simulink model "gm_sampleModel1853_5_sub"  (R2023a)
settings: Solver=VariableStepAuto  StartTime=0.0  StopTime=10.0  RelTol=1e-3
libraries: simulink x3, hdlsllib x2
settings Model: Creator=user1  LastModifiedBy=user1
settings OptimizationCC: BlockReduction=off  ConditionallyExecuteInputs=off
settings DebuggingCC: InheritedTsInSrcMsg=none

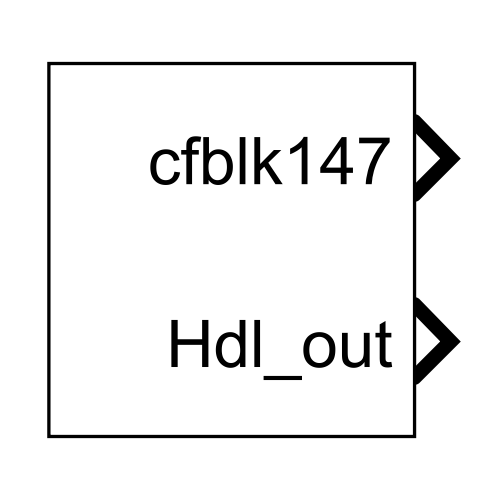
[thumbnail: Simulink's stored preview of the top-level diagram]
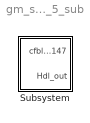
== system gm_sampleModel1853_5_sub ==
  Subsystem : Subsystem

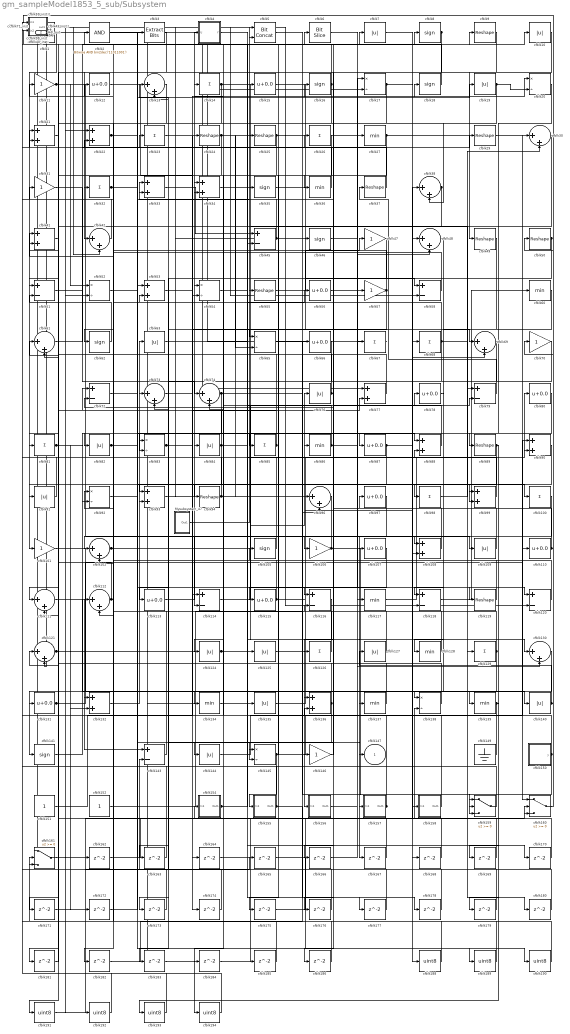
== system gm_sampleModel1853_5_sub/Subsystem ==
  Mysubsystem_47 : Subsystem
  cfblk1 : simulink/Logic and Bit Operations/Detect Increase  vinit=0.0  OutDataTypeStr=uint8
      settings: LibrarySourceBlock=|
      | hdlsllib/Logic and Bit
      | Operations/Detect
      | Increase
  cfblk{7,10,19,63,76,82,84,91,109,124..125,127,135,140,144} (15 alike) : Abs  OutDataTypeStr=uint8  SaturateOnIntegerOverflow=off
  cfblk{14,23,26,32,67..68,81,85,98,100,126,129} (12 alike) : Sum  Inputs=+  OutDataTypeStr=uint8
  cfblk{11,31,47,57,70,101,106,146} (8 alike) : Gain  OutDataTypeStr=uint8
  cfblk{13,30,38,42,48,61,69,73..74,96,102,111..112,121,130} (15 alike) : Sum  Inputs=|++  OutDataTypeStr=uint8
  cfblk103_inst : Subsystem
  cfblk104_inst : Subsystem
  cfblk{8,16,18,35,46,62,105,141} (8 alike) : Signum
  cfblk{12,15,56,66,78,80,87,97,107,110,113,115,131} (13 alike) : Bias  Bias=0.0  SaturateOnIntegerOverflow=off
  cfblk{21..22,33..34,41,53,77,88,90,93,99,108,132,136} (14 alike) : Sum  OutDataTypeStr=uint8
  cfblk{45,51,58,72,79,114,116,118,120,143} (10 alike) : Sum  Inputs=+-  OutDataTypeStr=uint8
  cfblk{27,36,60,86,117,128,134,137,139} (9 alike) : MinMax  OutDataTypeStr=uint8
  cfblk{9,24..25,29,37,49..50,55,89,94,119} (11 alike) : Reshape
  cfblk122_inst : Subsystem
  cfblk123_inst : Subsystem
  cfblk133_inst : Subsystem
  cfblk{17,20,52,54,65,83,92,138,145} (9 alike) : Product  Inputs=*/  OutDataTypeStr=uint8  RndMeth=Zero  SaturateOnIntegerOverflow=on
  cfblk142_inst : Subsystem
  cfblk149 : Ground
  cfblk150 : Subsystem  mask(Counter Limited){uplimit=double(7), tsamp=double(-1)}
      mask prompts: uplimit "Simulink:masks:UpperLimit_MP"; tsamp "Simulink:masks:SampleTime_MP"
      mask help: Simulink:masks:CounterLimited_MD
      mask init:
      | nbits = double(8);
      | tsamp = double(-1);
      | uplimit = double(7);
  cfblk151 : Constant  OutDataTypeStr=uint8  SampleTime=-1
  cfblk152 : Constant  OutDataTypeStr=uint8  SampleTime=-1
  cfblk154 : Subsystem
  cfblk155 : Subsystem
  cfblk156 : Subsystem
  cfblk157 : Subsystem
  cfblk158 : Subsystem
  cfblk159 : Switch  OutDataTypeStr=uint8  SaturateOnIntegerOverflow=off  InputSameDT=off
  cfblk160 : Switch  OutDataTypeStr=uint8  SaturateOnIntegerOverflow=off  InputSameDT=off
  cfblk161 : Switch  OutDataTypeStr=uint8  SaturateOnIntegerOverflow=off  InputSameDT=off
  cfblk{162..186} (25 alike) : Delay  SampleTime=1
  cfblk{188..194} (7 alike) : DataTypeConversion  OutDataTypeStr=uint8  SaturateOnIntegerOverflow=off  RndMeth=Floor
  cfblk2 : simulink/Logic and Bit Operations/Bitwise Operator  logicop=AND  UseBitMask=on  BitMask=bin2dec('11011001')  BitMaskRealWorld=Stored Integer
      settings: LibrarySourceBlock=|
      | hdlsllib/Logic and Bit
      | Operations/Bitwise
      | Operator
  cfblk28_inst : Subsystem
  cfblk3 : simulink/Logic and Bit Operations/Extract Bits  bitsToExtract=Upper half  numBits=8  bitIdxRange=[0 7]  outScalingMode=Preserve fixed-point scaling
      settings: LibrarySourceBlock=|
      | hdlsllib/Logic and Bit
      | Operations/Extract Bits
  cfblk39_inst : Subsystem
  cfblk4 : Subsystem  mask(Detect Fall Nonpositive){vinit=double(0), InputProcessing=Elements as channels (sample based), OutDataTypeStr=uint8}
      mask prompts: vinit "Simulink:masks:InitialCondition_MP"; InputProcessing "Simulink:masks:InputProcessing_MP"; OutDataTypeStr "Simulink:masks:OutputDataType_MP"
      mask help: Simulink:masks:DetectFallNonpositive_MD
      mask init:
      | InputProcessing = 'Elements as channels (sample based)';
      | OutDataTypeStr = 'uint8';
      | vinit = double(0);
      mask TypeOptions InputProcessing: Simulink:masks:ColumnsAsChannelsFrameBased | Simulink:masks:ElementsAsChannelsSampleBased
      mask TypeOptions OutDataTypeStr: Simulink:masks:uint8 | Simulink:masks:boolean
      mask Display: fprintf('U <= 0\n&  NOT\nU/z <= 0')
  cfblk40_inst : Subsystem
  cfblk43_inst : Subsystem
  cfblk5 : hdlsllib/Logic and Bit Operations/Bit Concat  numInputs=2
  cfblk59_inst : Subsystem
  cfblk6 : hdlsllib/Logic and Bit Operations/Bit Slice  lidx=7  ridx=0
  cfblk71_inst : Subsystem
  cfblk95_inst : Subsystem
  cfblk147 : Outport  OutDataTypeStr=uint8  SampleTime=1  VectorParamsAs1DForOutWhenUnconnected=off
  Hdl_out : Outport  Port=2  OutDataTypeStr=uint8
  wires:
  Mysubsystem_47/1(Out1) -> cfblk5/1
  cfblk1/1 -> cfblk101/1
  cfblk10/1 -> cfblk49/1
  cfblk100/1 -> cfblk167/1
  cfblk101/1 -> cfblk139/1
  cfblk102/1 -> cfblk76/1, cfblk120/1
  cfblk103_inst/1(out1) -> cfblk42/2, cfblk135/1
  cfblk104_inst/1(out1) -> cfblk125/1
  cfblk105/1 -> cfblk63/1
  cfblk106/1 -> cfblk159/3, cfblk102/1
  cfblk107/1 -> cfblk145/2
  cfblk108/1 -> cfblk97/1
  cfblk109/1 -> cfblk33/1
  cfblk11/1 -> cfblk114/2, cfblk52/1
  cfblk110/1 -> cfblk95_inst/1(in1), cfblk72/2, cfblk107/1
  cfblk111/1 -> cfblk143/1
  cfblk112/1 -> cfblk61/1, cfblk92/1
  cfblk113/1 -> cfblk4/1(U)
  cfblk114/1 -> cfblk78/1
  cfblk115/1 -> cfblk88/2, cfblk11/1
  cfblk116/1 -> cfblk156/1(In1)
  cfblk117/1 -> cfblk80/1
  cfblk118/1 -> cfblk60/1
  cfblk119/1 -> cfblk53/2
  cfblk12/1 -> cfblk174/1
  cfblk120/1 -> cfblk41/1
  cfblk121/1 -> cfblk66/1, cfblk132/2
  cfblk122_inst/1(out1) -> cfblk77/1, cfblk58/2
  cfblk123_inst/1(out1) -> cfblk96/1
  cfblk124/1 -> cfblk90/2, cfblk18/1
  cfblk125/1 -> cfblk68/1
  cfblk126/1 -> cfblk54/1
  cfblk127/1 -> cfblk84/1, cfblk21/1
  cfblk128/1 -> cfblk114/1
  cfblk129/1 -> cfblk157/1(In1), cfblk23/1
  cfblk13/1 -> cfblk191/1
  cfblk130/1 -> cfblk141/1
  cfblk131/1 -> cfblk90/1, cfblk3/1
  cfblk132/1 -> cfblk73/1
  cfblk133_inst/1(out1) -> cfblk30/1
  cfblk134/1 -> cfblk20/1
  cfblk135/1 -> cfblk57/1
  cfblk136/1 -> cfblk93/2, cfblk173/1
  cfblk137/1 -> cfblk122_inst/2(in2)
  cfblk138/1 -> cfblk6/1
  cfblk139/1 -> cfblk193/1, cfblk136/2
  cfblk14/1 -> cfblk42/1, cfblk137/1
  cfblk140/1 -> cfblk127/1, cfblk70/1
  cfblk141/1 -> cfblk112/1
  cfblk142_inst/1(out1) -> cfblk161/1, cfblk52/2
  cfblk143/1 -> cfblk28_inst/1(in1)
  cfblk144/1 -> cfblk110/1
  cfblk145/1 -> cfblk38/1, cfblk105/1, cfblk155/1(In1)
  cfblk146/1 -> cfblk86/1
  cfblk149/1 -> cfblk71_inst/2(in2)
  cfblk15/1 -> cfblk58/1
  cfblk150/1(y) -> cfblk5/2, cfblk159/2, cfblk116/2
  cfblk151/1 -> cfblk24/1
  cfblk152/1 -> cfblk45/2
  cfblk154/1(Out1) -> cfblk8/1, cfblk16/1, cfblk10/1
  cfblk155/1(Out1) -> cfblk43_inst/2(in2), cfblk177/1
  cfblk156/1(Out1) -> cfblk117/1
  cfblk157/1(Out1) -> cfblk74/2, cfblk13/1
  cfblk158/1(Out1) -> cfblk55/1
  cfblk159/1 -> cfblk122_inst/1(in1)
  cfblk16/1 -> cfblk132/1, cfblk103_inst/1(in1)
  cfblk160/1 -> cfblk50/1
  cfblk161/1 -> cfblk154/1(In1)
  cfblk162/1 -> cfblk160/2
  cfblk163/1 -> cfblk142_inst/2(in2)
  cfblk164/1 -> cfblk17/1
  cfblk165/1 -> cfblk190/1
  cfblk166/1 -> cfblk130/2
  cfblk167/1 -> cfblk111/2
  cfblk168/1 -> cfblk73/2
  cfblk169/1 -> cfblk121/1
  cfblk17/1 -> cfblk69/2, cfblk146/1
  cfblk170/1 -> cfblk138/2
  cfblk171/1 -> cfblk160/3
  cfblk172/1 -> cfblk34/1
  cfblk173/1 -> cfblk28_inst/2(in2)
  cfblk174/1 -> cfblk53/1
  cfblk175/1 -> cfblk118/2
  cfblk176/1 -> cfblk112/2
  cfblk177/1 -> cfblk33/2
  cfblk178/1 -> cfblk143/2
  cfblk179/1 -> cfblk40_inst/2(in2)
  cfblk18/1 -> cfblk133_inst/2(in2)
  cfblk180/1 -> cfblk161/2
  cfblk181/1 -> cfblk61/2
  cfblk182/1 -> cfblk96/2
  cfblk183/1 -> cfblk194/1
  cfblk184/1 -> cfblk48/1
  cfblk185/1 -> cfblk102/2
  cfblk186/1 -> cfblk161/3
  cfblk188/1 -> cfblk2/1
  cfblk189/1 -> cfblk71_inst/1(in1)
  cfblk19/1 -> cfblk82/1, cfblk38/2, cfblk20/2
  cfblk190/1 -> cfblk123_inst/2(in2)
  cfblk191/1 -> cfblk165/1
  cfblk192/1 -> cfblk123_inst/1(in1)
  cfblk193/1 -> cfblk39_inst/1(in1)
  cfblk194/1 -> cfblk39_inst/2(in2)
  cfblk2/1 -> cfblk189/1
  cfblk20/1 -> cfblk89/1
  cfblk21/1 -> cfblk181/1
  cfblk22/1 -> cfblk9/1, cfblk19/1
  cfblk23/1 -> cfblk164/1
  cfblk24/1 -> cfblk188/1, cfblk65/2, cfblk54/2
  cfblk25/1 -> cfblk51/1, cfblk111/1
  cfblk26/1 -> cfblk144/1
  cfblk27/1 -> cfblk65/1, cfblk166/1
  cfblk28_inst/1(out1) -> cfblk121/2, cfblk120/2, cfblk185/1
  cfblk29/1 -> cfblk160/1
  cfblk3/1 -> cfblk32/1
  cfblk30/1 -> cfblk81/1
  cfblk31/1 -> cfblk74/1
  cfblk32/1 -> cfblk87/1, cfblk147/1
  cfblk33/1 -> cfblk45/1
  cfblk34/1 -> cfblk129/1
  cfblk35/1 -> cfblk168/1
  cfblk36/1 -> cfblk40_inst/1(in1)
  cfblk37/1 -> cfblk14/1
  cfblk38/1 -> cfblk62/1, cfblk175/1
  cfblk39_inst/1(out1) -> cfblk192/1
  cfblk4/1(Y) -> cfblk170/1
  cfblk40_inst/1(out1) -> cfblk17/2, cfblk162/1
  cfblk41/1 -> cfblk91/1
  cfblk42/1 -> cfblk104_inst/1(in1)
  cfblk43_inst/1(out1) -> cfblk27/1
  cfblk45/1 -> cfblk34/2, cfblk158/1(In1)
  cfblk46/1 -> cfblk67/1
  cfblk47/1 -> cfblk93/1
  cfblk48/1 -> cfblk118/1
  cfblk49/1 -> cfblk108/1
  cfblk5/1 -> cfblk159/1
  cfblk50/1 -> cfblk115/1, cfblk85/1
  cfblk51/1 -> cfblk7/1
  cfblk52/1 -> cfblk108/2
  cfblk53/1 -> cfblk69/1
  cfblk54/1 -> cfblk130/1
  cfblk55/1 -> cfblk47/1
  cfblk56/1 -> cfblk109/1
  cfblk57/1 -> cfblk83/2, cfblk31/1
  cfblk58/1 -> cfblk12/1
  cfblk59_inst/1(out1) -> cfblk22/1
  cfblk6/1 -> cfblk119/1
  cfblk60/1 -> cfblk128/1
  cfblk61/1 -> cfblk29/1
  cfblk62/1 -> cfblk41/2
  cfblk63/1 -> cfblk178/1
  cfblk65/1 -> cfblk99/2
  cfblk66/1 -> cfblk163/1
  cfblk67/1 -> cfblk1/1
  cfblk68/1 -> cfblk22/2, cfblk124/1, cfblk180/1
  cfblk69/1 -> cfblk94/1
  cfblk7/1 -> cfblk99/1
  cfblk70/1 -> cfblk184/1
  cfblk71_inst/1(out1) -> cfblk46/1
  cfblk72/1 -> cfblk116/1
  cfblk73/1 -> cfblk140/1
  cfblk74/1 -> cfblk88/1, cfblk92/2
  cfblk76/1 -> cfblk59_inst/2(in2), cfblk126/1
  cfblk77/1 -> cfblk13/2
  cfblk78/1 -> cfblk138/1
  cfblk79/1 -> cfblk37/1
  cfblk8/1 -> cfblk131/1, cfblk36/1
  cfblk80/1 -> cfblk83/1
  cfblk81/1 -> cfblk136/1, cfblk172/1
  cfblk82/1 -> cfblk35/1, cfblk100/1
  cfblk83/1 -> cfblk77/2, cfblk98/1
  cfblk84/1 -> cfblk79/2, cfblk56/1, cfblk21/2, cfblk183/1, cfblk182/1
  cfblk85/1 -> cfblk95_inst/2(in2), cfblk72/1, cfblk142_inst/1(in1)
  cfblk86/1 -> cfblk48/2, cfblk104_inst/2(in2)
  cfblk87/1 -> cfblk79/1, cfblk186/1
  cfblk88/1 -> cfblk26/1
  cfblk89/1 -> cfblk113/1, cfblk171/1, cfblk169/1
  cfblk9/1 -> cfblk176/1
  cfblk90/1 -> cfblk179/1
  cfblk91/1 -> cfblk133_inst/1(in1)
  cfblk92/1 -> cfblk145/1
  cfblk93/1 -> cfblk15/1
  cfblk94/1 -> cfblk51/2, cfblk25/1, cfblk103_inst/2(in2)
  cfblk95_inst/1(out1) -> cfblk43_inst/1(in1)
  cfblk96/1 -> cfblk106/1
  cfblk97/1 -> cfblk134/1
  cfblk98/1 -> cfblk30/2
  cfblk99/1 -> cfblk59_inst/1(in1)

== system gm_sampleModel1853_5_sub/Subsystem/Mysubsystem_47 ==
  cfblk153 : Subsystem  mask(Counter Limited){uplimit=double(7), tsamp=double(-1)}
      mask prompts: uplimit "Simulink:masks:UpperLimit_MP"; tsamp "Simulink:masks:SampleTime_MP"
      mask help: Simulink:masks:CounterLimited_MD
      mask init:
      | nbits = double(8);
      | tsamp = double(-1);
      | uplimit = double(7);
  cfblk44 : Abs  SaturateOnIntegerOverflow=off
  Out1 : Outport  SampleTime=1
  wires:
  cfblk153/1(y) -> cfblk44/1
  cfblk44/1 -> Out1/1

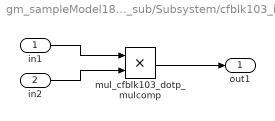
== system gm_sampleModel1853_5_sub/Subsystem/cfblk103_inst ==
  in1 : Inport  OutDataTypeStr=uint8  SampleTime=1
  in2 : Inport  Port=2  OutDataTypeStr=uint8  SampleTime=1
  mul_cfblk103_dotp_mulcomp : Product  Inputs=**  OutDataTypeStr=uint8  SampleTime=1
  out1 : Outport  OutDataTypeStr=uint8  SampleTime=1
  wires:
  in1/1 -> mul_cfblk103_dotp_mulcomp/1
  in2/1 -> mul_cfblk103_dotp_mulcomp/2
  mul_cfblk103_dotp_mulcomp/1 -> out1/1

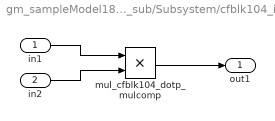
== system gm_sampleModel1853_5_sub/Subsystem/cfblk104_inst ==
  in1 : Inport  OutDataTypeStr=uint8  SampleTime=1
  in2 : Inport  Port=2  OutDataTypeStr=uint8  SampleTime=1
  mul_cfblk104_dotp_mulcomp : Product  Inputs=**  OutDataTypeStr=uint8  SampleTime=1
  out1 : Outport  OutDataTypeStr=uint8  SampleTime=1
  wires:
  in1/1 -> mul_cfblk104_dotp_mulcomp/1
  in2/1 -> mul_cfblk104_dotp_mulcomp/2
  mul_cfblk104_dotp_mulcomp/1 -> out1/1

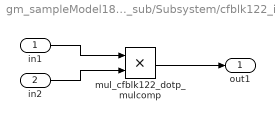
== system gm_sampleModel1853_5_sub/Subsystem/cfblk122_inst ==
  in1 : Inport  OutDataTypeStr=uint8  SampleTime=1
  in2 : Inport  Port=2  OutDataTypeStr=uint8  SampleTime=1
  mul_cfblk122_dotp_mulcomp : Product  Inputs=**  OutDataTypeStr=uint8  SampleTime=1
  out1 : Outport  OutDataTypeStr=uint8  SampleTime=1
  wires:
  in1/1 -> mul_cfblk122_dotp_mulcomp/1
  in2/1 -> mul_cfblk122_dotp_mulcomp/2
  mul_cfblk122_dotp_mulcomp/1 -> out1/1

== system gm_sampleModel1853_5_sub/Subsystem/cfblk123_inst ==
  in1 : Inport  OutDataTypeStr=uint8  SampleTime=1
  in2 : Inport  Port=2  OutDataTypeStr=uint8  SampleTime=1
  mul_cfblk123_dotp_mulcomp : Product  Inputs=**  OutDataTypeStr=uint8  SampleTime=1
  out1 : Outport  OutDataTypeStr=uint8  SampleTime=1
  wires:
  in1/1 -> mul_cfblk123_dotp_mulcomp/1
  in2/1 -> mul_cfblk123_dotp_mulcomp/2
  mul_cfblk123_dotp_mulcomp/1 -> out1/1

== system gm_sampleModel1853_5_sub/Subsystem/cfblk133_inst ==
  in1 : Inport  OutDataTypeStr=uint8  SampleTime=1
  in2 : Inport  Port=2  OutDataTypeStr=uint8  SampleTime=1
  mul_cfblk133_dotp_mulcomp : Product  Inputs=**  OutDataTypeStr=uint8  SampleTime=1
  out1 : Outport  OutDataTypeStr=uint8  SampleTime=1
  wires:
  in1/1 -> mul_cfblk133_dotp_mulcomp/1
  in2/1 -> mul_cfblk133_dotp_mulcomp/2
  mul_cfblk133_dotp_mulcomp/1 -> out1/1

== system gm_sampleModel1853_5_sub/Subsystem/cfblk142_inst ==
  in1 : Inport  OutDataTypeStr=uint8  SampleTime=1
  in2 : Inport  Port=2  OutDataTypeStr=uint8  SampleTime=1
  mul_cfblk142_dotp_mulcomp : Product  Inputs=**  OutDataTypeStr=uint8  SampleTime=1
  out1 : Outport  OutDataTypeStr=uint8  SampleTime=1
  wires:
  in1/1 -> mul_cfblk142_dotp_mulcomp/1
  in2/1 -> mul_cfblk142_dotp_mulcomp/2
  mul_cfblk142_dotp_mulcomp/1 -> out1/1

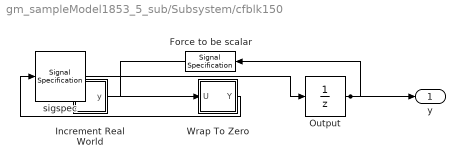
== system gm_sampleModel1853_5_sub/Subsystem/cfblk150 ==
  Force to be scalar : SignalSpecification  DisableCoverage=on  Dimensions=1
  Increment Real World : Subsystem  mask(Real World Value Increment){}
      mask help: Simulink:masks:RealWorldValueIncrement_MD
      mask Display: disp('V++')
  Output : UnitDelay  InitialCondition=0.0  SampleTime=tsamp  HasFrameUpgradeWarning=on
  Wrap To Zero : Subsystem  mask(Wrap To Zero){Threshold=double(7)}
      mask prompts: Threshold "Simulink:masks:Threshold_MP"
      mask help: Simulink:masks:WrapToZero_MD
  sigspec : SignalSpecification  OutDataTypeStr=uint8  Dimensions=1
  y : Outport  SampleTime=1
  wires:
  Force to be scalar/1 -> Increment Real World/1(u)
  Increment Real World/1(y) -> Wrap To Zero/1(U)
  Output/1 -> Force to be scalar/1, y/1
  Wrap To Zero/1(Y) -> sigspec/1
  sigspec/1 -> Output/1

== system gm_sampleModel1853_5_sub/Subsystem/cfblk154 ==
  In1 : Inport  OutDataTypeStr=uint8  PortDimensions=1  SampleTime=1
  Out1 : Outport  SampleTime=1
  wires:
  In1/1 -> Out1/1

== system gm_sampleModel1853_5_sub/Subsystem/cfblk155 ==
  In1 : Inport  OutDataTypeStr=uint8  PortDimensions=1  SampleTime=1
  Out1 : Outport  SampleTime=1
  wires:
  In1/1 -> Out1/1

== system gm_sampleModel1853_5_sub/Subsystem/cfblk156 ==
  In1 : Inport  OutDataTypeStr=uint8  PortDimensions=1  SampleTime=1
  Out1 : Outport  SampleTime=1
  wires:
  In1/1 -> Out1/1

== system gm_sampleModel1853_5_sub/Subsystem/cfblk157 ==
  In1 : Inport  OutDataTypeStr=uint8  PortDimensions=1  SampleTime=1
  Out1 : Outport  SampleTime=1
  wires:
  In1/1 -> Out1/1

== system gm_sampleModel1853_5_sub/Subsystem/cfblk158 ==
  In1 : Inport  OutDataTypeStr=uint8  PortDimensions=1  SampleTime=1
  Out1 : Outport  SampleTime=1
  wires:
  In1/1 -> Out1/1

== system gm_sampleModel1853_5_sub/Subsystem/cfblk28_inst ==
  in1 : Inport  OutDataTypeStr=uint8  SampleTime=1
  in2 : Inport  Port=2  OutDataTypeStr=uint8  SampleTime=1
  mul_cfblk28_dotp_mulcomp : Product  Inputs=**  OutDataTypeStr=uint8  SampleTime=1
  out1 : Outport  OutDataTypeStr=uint8  SampleTime=1
  wires:
  in1/1 -> mul_cfblk28_dotp_mulcomp/1
  in2/1 -> mul_cfblk28_dotp_mulcomp/2
  mul_cfblk28_dotp_mulcomp/1 -> out1/1

== system gm_sampleModel1853_5_sub/Subsystem/cfblk39_inst ==
  in1 : Inport  OutDataTypeStr=uint8  SampleTime=1
  in2 : Inport  Port=2  OutDataTypeStr=uint8  SampleTime=1
  mul_cfblk39_dotp_mulcomp : Product  Inputs=**  OutDataTypeStr=uint8  SampleTime=1
  out1 : Outport  OutDataTypeStr=uint8  SampleTime=1
  wires:
  in1/1 -> mul_cfblk39_dotp_mulcomp/1
  in2/1 -> mul_cfblk39_dotp_mulcomp/2
  mul_cfblk39_dotp_mulcomp/1 -> out1/1

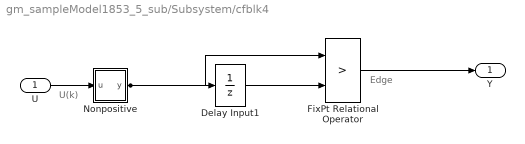
== system gm_sampleModel1853_5_sub/Subsystem/cfblk4 ==
  note: U(k)
  note: Edge
  U : Inport  OutDataTypeStr=uint8  SampleTime=1
  Delay Input1 : UnitDelay  Description=Store in Global RAM  DisableCoverage=on  InitialCondition=vinit  SampleTime=-1  HasFrameUpgradeWarning=on
  FixPt Relational Operator : RelationalOperator  Operator=>  OutDataTypeStr=fixdt(0, 8)  ZeroCross=off  InputSameDT=off
  Nonpositive : Subsystem  mask(Compare To Zero){relop=<=, OutDataTypeStr=boolean, ZeroCross=off}
      mask prompts: relop "Simulink:masks:Operator_MP"; OutDataTypeStr "Simulink:masks:OutputDataType_MP"; ZeroCross "Simulink:masks:EnableZerocrossingDetection_MP"
      mask help: Simulink:masks:CompareToZero_MD
      mask init:
      | OutDataTypeStr = 'boolean';
      | ZeroCross = 'off';
      | blkName = 'sampleModel1853_5_sub/Subsystem/cfblk4/Nonpositive';
      | relop = '<=';
      | setValue = 'boolean';
      mask TypeOptions relop: == | ~= | < | <= | >= | >
      mask TypeOptions OutDataTypeStr: Simulink:masks:uint8 | Simulink:masks:boolean
      mask Callback ZeroCross: sl('zeroCrossEnable', gcbh);
      mask Display: disp([relop,' 0'])
  Y : Outport  SampleTime=1
  wires:
  U/1 -> Nonpositive/1(u)
  Delay Input1/1 -> FixPt Relational Operator/2
  FixPt Relational Operator/1 -> Y/1
  Nonpositive/1(y) -> FixPt Relational Operator/1, Delay Input1/1

== system gm_sampleModel1853_5_sub/Subsystem/cfblk40_inst ==
  in1 : Inport  OutDataTypeStr=uint8  SampleTime=1
  in2 : Inport  Port=2  OutDataTypeStr=uint8  SampleTime=1
  mul_cfblk40_dotp_mulcomp : Product  Inputs=**  OutDataTypeStr=uint8  SampleTime=1
  out1 : Outport  OutDataTypeStr=uint8  SampleTime=1
  wires:
  in1/1 -> mul_cfblk40_dotp_mulcomp/1
  in2/1 -> mul_cfblk40_dotp_mulcomp/2
  mul_cfblk40_dotp_mulcomp/1 -> out1/1

== system gm_sampleModel1853_5_sub/Subsystem/cfblk43_inst ==
  in1 : Inport  OutDataTypeStr=uint8  SampleTime=1
  in2 : Inport  Port=2  OutDataTypeStr=uint8  SampleTime=1
  mul_cfblk43_dotp_mulcomp : Product  Inputs=**  OutDataTypeStr=uint8  SampleTime=1
  out1 : Outport  OutDataTypeStr=uint8  SampleTime=1
  wires:
  in1/1 -> mul_cfblk43_dotp_mulcomp/1
  in2/1 -> mul_cfblk43_dotp_mulcomp/2
  mul_cfblk43_dotp_mulcomp/1 -> out1/1

== system gm_sampleModel1853_5_sub/Subsystem/cfblk59_inst ==
  in1 : Inport  OutDataTypeStr=uint8  SampleTime=1
  in2 : Inport  Port=2  OutDataTypeStr=uint8  SampleTime=1
  mul_cfblk59_dotp_mulcomp : Product  Inputs=**  OutDataTypeStr=uint8  SampleTime=1
  out1 : Outport  OutDataTypeStr=uint8  SampleTime=1
  wires:
  in1/1 -> mul_cfblk59_dotp_mulcomp/1
  in2/1 -> mul_cfblk59_dotp_mulcomp/2
  mul_cfblk59_dotp_mulcomp/1 -> out1/1

== system gm_sampleModel1853_5_sub/Subsystem/cfblk71_inst ==
  in1 : Inport  OutDataTypeStr=uint8  SampleTime=1
  in2 : Inport  Port=2  OutDataTypeStr=uint8
  mul_cfblk71_dotp_mulcomp : Product  Inputs=**  OutDataTypeStr=uint8  SampleTime=1
  out1 : Outport  OutDataTypeStr=uint8  SampleTime=1
  wires:
  in1/1 -> mul_cfblk71_dotp_mulcomp/1
  in2/1 -> mul_cfblk71_dotp_mulcomp/2
  mul_cfblk71_dotp_mulcomp/1 -> out1/1

== system gm_sampleModel1853_5_sub/Subsystem/cfblk95_inst ==
  in1 : Inport  OutDataTypeStr=uint8  SampleTime=1
  in2 : Inport  Port=2  OutDataTypeStr=uint8  SampleTime=1
  mul_cfblk95_dotp_mulcomp : Product  Inputs=**  OutDataTypeStr=uint8  SampleTime=1
  out1 : Outport  OutDataTypeStr=uint8  SampleTime=1
  wires:
  in1/1 -> mul_cfblk95_dotp_mulcomp/1
  in2/1 -> mul_cfblk95_dotp_mulcomp/2
  mul_cfblk95_dotp_mulcomp/1 -> out1/1

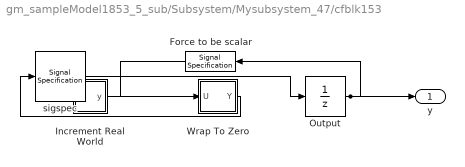
== system gm_sampleModel1853_5_sub/Subsystem/Mysubsystem_47/cfblk153 ==
  Force to be scalar : SignalSpecification  DisableCoverage=on  Dimensions=1
  Increment Real World : Subsystem  mask(Real World Value Increment){}
      mask help: Simulink:masks:RealWorldValueIncrement_MD
      mask Display: disp('V++')
  Output : UnitDelay  InitialCondition=0.0  SampleTime=tsamp  HasFrameUpgradeWarning=on
  Wrap To Zero : Subsystem  mask(Wrap To Zero){Threshold=double(7)}
      mask prompts: Threshold "Simulink:masks:Threshold_MP"
      mask help: Simulink:masks:WrapToZero_MD
  sigspec : SignalSpecification  OutDataTypeStr=uint8  Dimensions=1
  y : Outport  SampleTime=1
  wires:
  Force to be scalar/1 -> Increment Real World/1(u)
  Increment Real World/1(y) -> Wrap To Zero/1(U)
  Output/1 -> Force to be scalar/1, y/1
  Wrap To Zero/1(Y) -> sigspec/1
  sigspec/1 -> Output/1

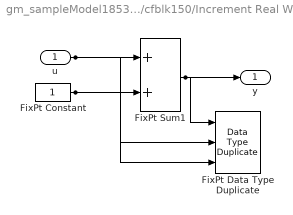
== system gm_sampleModel1853_5_sub/Subsystem/cfblk150/Increment Real World ==
  u : Inport  OutDataTypeStr=uint8  SampleTime=1
  FixPt Constant : Constant  DisableCoverage=on  OutDataTypeStr=Inherit: Inherit via back propagation  SampleTime=-1
  FixPt Data Type Duplicate : DataTypeDuplicate  DisableCoverage=on  NumInputPorts=3
  FixPt Sum1 : Sum  InputSameDT=on  OutDataTypeStr=Inherit: Inherit via back propagation  LockScale=on
  y : Outport  SampleTime=1
  wires:
  u/1 -> FixPt Sum1/1, FixPt Data Type Duplicate/2
  FixPt Constant/1 -> FixPt Sum1/2, FixPt Data Type Duplicate/3
  FixPt Sum1/1 -> FixPt Data Type Duplicate/1, y/1

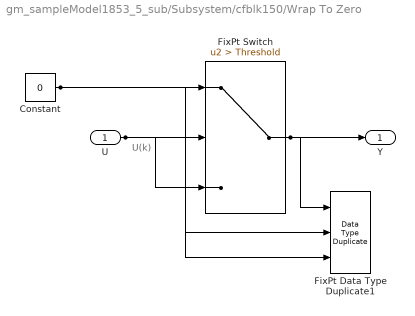
== system gm_sampleModel1853_5_sub/Subsystem/cfblk150/Wrap To Zero ==
  note: U(k)
  U : Inport  OutDataTypeStr=uint8  SampleTime=1
  Constant : Constant  DisableCoverage=on  Value=0  OutDataTypeStr=Inherit: Inherit via back propagation  SampleTime=-1
  FixPt Data Type Duplicate1 : DataTypeDuplicate  DisableCoverage=on  NumInputPorts=3
  FixPt Switch : Switch  Criteria=u2 > Threshold  Threshold=Threshold  OutDataTypeStr=Inherit: Inherit via back propagation  ZeroCross=off  SaturateOnIntegerOverflow=off  InputSameDT=off
  Y : Outport  SampleTime=1
  wires:
  U/1 -> FixPt Switch/3, FixPt Switch/2, FixPt Data Type Duplicate1/2
  Constant/1 -> FixPt Switch/1, FixPt Data Type Duplicate1/3
  FixPt Switch/1 -> FixPt Data Type Duplicate1/1, Y/1

== system gm_sampleModel1853_5_sub/Subsystem/cfblk4/Nonpositive ==
  u : Inport  OutDataTypeStr=uint8  SampleTime=1
  Compare : RelationalOperator  Operator=<=  OutDataTypeStr=boolean  ZeroCross=off
  Constant : Constant  DisableCoverage=on  Value=0  OutDataTypeStr=Inherit: Inherit via back propagation  SampleTime=-1  PreserveConstantTs=on
  y : Outport  SampleTime=1
  wires:
  u/1 -> Compare/1
  Compare/1 -> y/1
  Constant/1 -> Compare/2

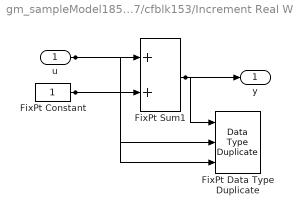
== system gm_sampleModel1853_5_sub/Subsystem/Mysubsystem_47/cfblk153/Increment Real World ==
  u : Inport  OutDataTypeStr=uint8  SampleTime=1
  FixPt Constant : Constant  DisableCoverage=on  OutDataTypeStr=Inherit: Inherit via back propagation  SampleTime=-1
  FixPt Data Type Duplicate : DataTypeDuplicate  DisableCoverage=on  NumInputPorts=3
  FixPt Sum1 : Sum  InputSameDT=on  OutDataTypeStr=Inherit: Inherit via back propagation  LockScale=on
  y : Outport  SampleTime=1
  wires:
  u/1 -> FixPt Sum1/1, FixPt Data Type Duplicate/2
  FixPt Constant/1 -> FixPt Sum1/2, FixPt Data Type Duplicate/3
  FixPt Sum1/1 -> FixPt Data Type Duplicate/1, y/1

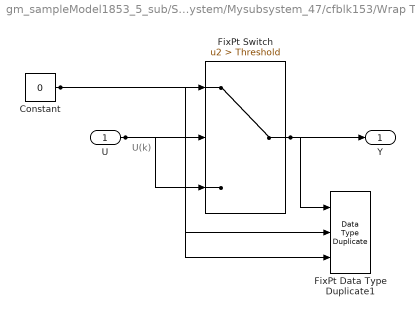
== system gm_sampleModel1853_5_sub/Subsystem/Mysubsystem_47/cfblk153/Wrap To Zero ==
  note: U(k)
  U : Inport  OutDataTypeStr=uint8  SampleTime=1
  Constant : Constant  DisableCoverage=on  Value=0  OutDataTypeStr=Inherit: Inherit via back propagation  SampleTime=-1
  FixPt Data Type Duplicate1 : DataTypeDuplicate  DisableCoverage=on  NumInputPorts=3
  FixPt Switch : Switch  Criteria=u2 > Threshold  Threshold=Threshold  OutDataTypeStr=Inherit: Inherit via back propagation  ZeroCross=off  SaturateOnIntegerOverflow=off  InputSameDT=off
  Y : Outport  SampleTime=1
  wires:
  U/1 -> FixPt Switch/3, FixPt Switch/2, FixPt Data Type Duplicate1/2
  Constant/1 -> FixPt Switch/1, FixPt Data Type Duplicate1/3
  FixPt Switch/1 -> FixPt Data Type Duplicate1/1, Y/1
